simulink model "cvicenie_2"  (R2024b)
settings: Solver=VariableStepAuto  StartTime=0.0  StopTime=9  RelTol=1e-3
values from neighbouring files (symbols this model uses):
  omega_0 = 2*pi*(1/T)    (= 1.3962634016)    [cvicenie_2_omega.m]
settings Model: Creator=Nergigante  LastModifiedBy=Nergigante

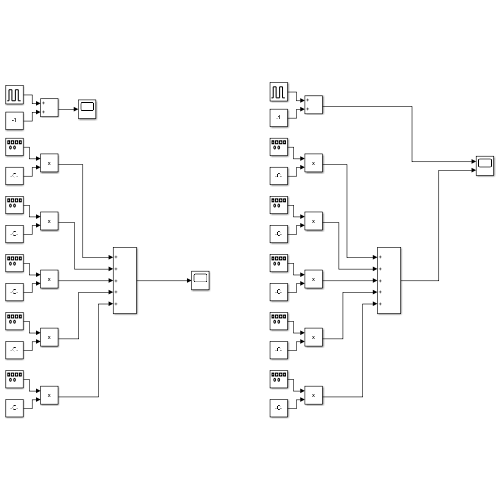
[thumbnail: Simulink's stored preview of the top-level diagram]
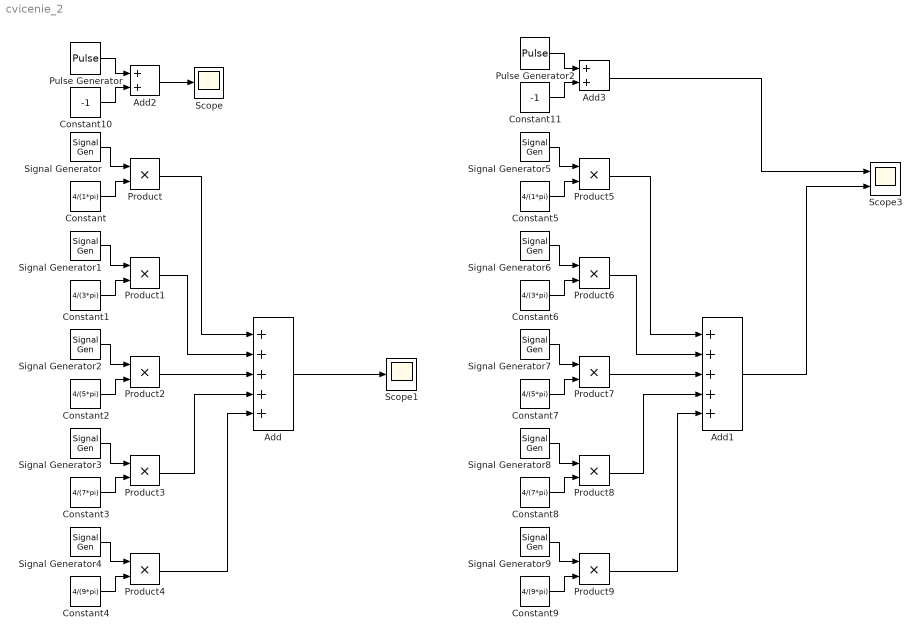
== system cvicenie_2 ==
  Add : Sum  Inputs=+++++
  Add1 : Sum  Inputs=+++++
  Add2 : Sum
  Add3 : Sum
  Constant : Constant  Value=4/(1*pi)
  Constant1 : Constant  Value=4/(3*pi)
  Constant10 : Constant  Value=-1
  Constant11 : Constant  Value=-1
  Constant2 : Constant  Value=4/(5*pi)
  Constant3 : Constant  Value=4/(7*pi)
  Constant4 : Constant  Value=4/(9*pi)
  Constant5 : Constant  Value=4/(1*pi)
  Constant6 : Constant  Value=4/(3*pi)
  Constant7 : Constant  Value=4/(5*pi)
  Constant8 : Constant  Value=4/(7*pi)
  Constant9 : Constant  Value=4/(9*pi)
  Product{,1..9} (10 alike) : Product
  Pulse Generator : DiscretePulseGenerator  PulseType=Time based  Amplitude=2  Period=4.5  PulseWidth=50
  Pulse Generator2 : DiscretePulseGenerator  PulseType=Time based  Amplitude=2  Period=4.5  PulseWidth=50
  Scope : Scope
  Scope1 : Scope
  Scope3 : Scope  NumInputPorts=2
  Signal Generator : SignalGenerator  Frequency=omega_0  Units=rad/sec
  Signal Generator1 : SignalGenerator  Frequency=3*omega_0  Units=rad/sec
  Signal Generator2 : SignalGenerator  Frequency=5*omega_0  Units=rad/sec
  Signal Generator3 : SignalGenerator  Frequency=7*omega_0  Units=rad/sec
  Signal Generator4 : SignalGenerator  Frequency=9*omega_0  Units=rad/sec
  Signal Generator5 : SignalGenerator  Frequency=omega_0  Units=rad/sec
  Signal Generator6 : SignalGenerator  Frequency=3*omega_0  Units=rad/sec
  Signal Generator7 : SignalGenerator  Frequency=5*omega_0  Units=rad/sec
  Signal Generator8 : SignalGenerator  Frequency=7*omega_0  Units=rad/sec
  Signal Generator9 : SignalGenerator  Frequency=9*omega_0  Units=rad/sec
  wires:
  Signal Generator/1 -> Product/1
  Constant/1 -> Product/2
  Signal Generator1/1 -> Product1/1
  Constant1/1 -> Product1/2
  Signal Generator2/1 -> Product2/1
  Constant2/1 -> Product2/2
  Signal Generator3/1 -> Product3/1
  Constant3/1 -> Product3/2
  Signal Generator4/1 -> Product4/1
  Constant4/1 -> Product4/2
  Product1/1 -> Add/2
  Product3/1 -> Add/4
  Product2/1 -> Add/3
  Product/1 -> Add/1
  Product4/1 -> Add/5
  Add/1 -> Scope1/1
  Product5/1 -> Add1/1
  Product6/1 -> Add1/2
  Product7/1 -> Add1/3
  Product8/1 -> Add1/4
  Signal Generator6/1 -> Product6/1
  Signal Generator5/1 -> Product5/1
  Product9/1 -> Add1/5
  Constant8/1 -> Product8/2
  Signal Generator9/1 -> Product9/1
  Constant6/1 -> Product6/2
  Constant9/1 -> Product9/2
  Constant5/1 -> Product5/2
  Signal Generator8/1 -> Product8/1
  Signal Generator7/1 -> Product7/1
  Constant7/1 -> Product7/2
  Add1/1 -> Scope3/2
  Pulse Generator/1 -> Add2/1
  Constant10/1 -> Add2/2
  Add2/1 -> Scope/1
  Pulse Generator2/1 -> Add3/1
  Constant11/1 -> Add3/2
  Add3/1 -> Scope3/1
